simulink model "lqr_arduino_basic"  (R2015a)
settings: Solver=ode3  StartTime=0.0  StopTime=10.0  FixedStep=1/200  RelTol=1e-3
undefined symbols (not defined in the file or in its folder): Discrete, Hinf, Obs, Obs2, Time
libraries: PoliArd x8, ctrlSharedLib x2, simulink x1
settings Model: ExtModeTrigDuration=2  Creator=User  LastModifiedBy=user
settings OptimizationCC: OptimizeModelRefInitCode=on  LifeSpan=1
settings DebuggingCC: UnderspecifiedInitializationDetection=Classic  MergeDetectMultiDrivingBlocksExec=none
settings HardwareCC: ProdLargestAtomicInteger=Long  ProdLargestAtomicFloat=Double  ProdEndianess=LittleEndian  ProdHWDeviceType=ARM Compatible->ARM Cortex
settings RTWCC: SystemTargetFile=realtime.tlc  GenerateMakefile=off  TemplateMakefile=realtime.tmf  Description=Run on Target Hardware  RTWVerbose=off
settings ERTTargetCC: CombineOutputUpdateFcns=off  ExtModeTransport=3  ExtModeMexFile=ext_serial_win32_comm_rtt  ExtModeMexArgs=0 1 9600  ERTSrcFileBannerTemplate=realtime_code_template.cgt  ERTHdrFileBannerTemplate=realtime_code_template.cgt  ERTDataSrcFileTemplate=realtime_code_template.cgt  ERTDataHdrFileTemplate=realtime_code_template.cgt  ERTCustomFileTemplate=realtime_file_process.tlc

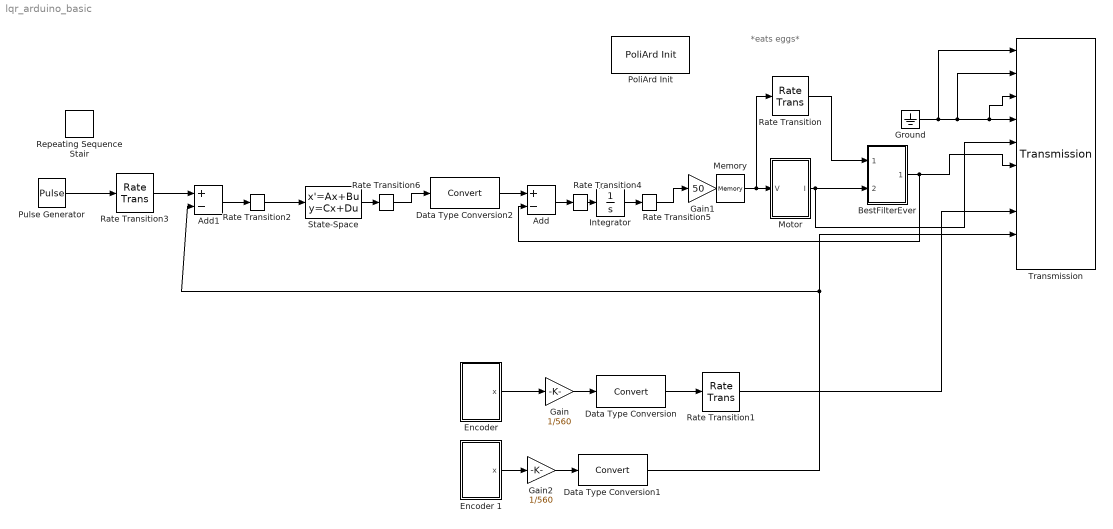
== system lqr_arduino_basic ==
  note: *eats eggs*
  Add : Sum  Inputs=+-
  Add1 : Sum  Inputs=+-
  BestFilterEver : Subsystem
  Data Type Conversion : DataTypeConversion
  Data Type Conversion1 : DataTypeConversion
  Data Type Conversion2 : DataTypeConversion
  "Encoder " : Subsystem
  Encoder 1 : Subsystem
  Gain : Gain  Gain=1/560
  Gain1 : Gain  Gain=50
  Gain2 : Gain  Gain=1/560
  Ground : Ground
  Integrator : Integrator
  Memory : Memory  InheritSampleTime=on
  Motor : Subsystem
  PoliArd Init : PoliArd/PoliArd Init
  Pulse Generator : DiscretePulseGenerator  PulseType=Time based  Amplitude=1.5  Period=7  PulseWidth=50  PhaseDelay=3
  Rate Transition{,1..6} (7 alike) : RateTransition
  Repeating Sequence Stair : simulink/Sources/Repeating Sequence Stair  OutValues=[1 2 -1 -2]  tsamp=5  OutMin=[]  OutMax=[]  OutDataTypeStr=double  OutputDataTypeScalingMode=double  OutDataType=fixdt(0,8)  ConRadixGroup=Best Precision: Vector-wise  OutScaling=2^-12
  State-Space : StateSpace  A=Hinf.A  B=Hinf.B  C=Hinf.C  D=Hinf.D  X0=0
  Transmission : PoliArd/Transmission  sample_freq=200  sig_to_send=6
  wires:
  Ground/1 -> Transmission/2, Transmission/3, Transmission/4, Transmission/1
  "Encoder "/1(x) -> Gain/1
  Gain/1 -> Data Type Conversion/1
  Data Type Conversion/1 -> Rate Transition1/1
  Encoder 1/1(x) -> Gain2/1
  Gain2/1 -> Data Type Conversion1/1
  Data Type Conversion1/1 -> Transmission/9, Add1/2
  Rate Transition1/1 -> Transmission/8
  Pulse Generator/1 -> Rate Transition3/1
  Motor/1(I) -> Transmission/5, BestFilterEver/2(In2)
  Rate Transition/1 -> BestFilterEver/1(In1)
  BestFilterEver/1(Out2) -> Add/2, Transmission/6
  Add/1 -> Rate Transition4/1
  Gain1/1 -> Memory/1
  Rate Transition5/1 -> Gain1/1
  Integrator/1 -> Rate Transition5/1
  Rate Transition4/1 -> Integrator/1
  Rate Transition3/1 -> Add1/1
  Add1/1 -> Rate Transition2/1
  Rate Transition2/1 -> State-Space/1
  State-Space/1 -> Rate Transition6/1
  Rate Transition6/1 -> Data Type Conversion2/1
  Data Type Conversion2/1 -> Add/1
  Memory/1 -> Rate Transition/1, Motor/1(V)

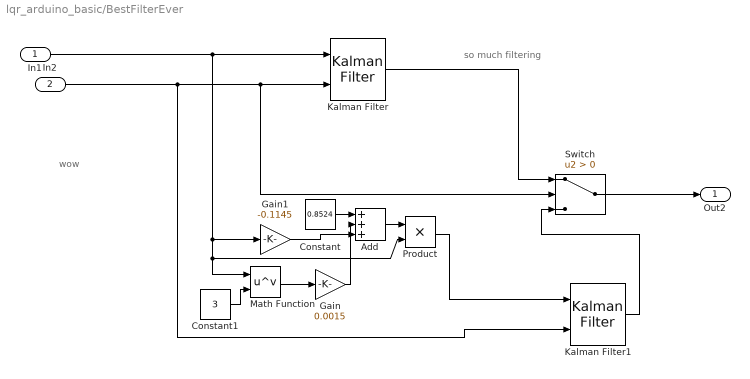
== system lqr_arduino_basic/BestFilterEver ==
  note: wow
  note: so much filtering
  In1 : Inport
  In2 : Inport  Port=2
  Add : Sum  Inputs=+++
  Constant : Constant  Value=0.8524
  Constant1 : Constant  Value=3
  Gain : Gain  Gain=0.0015
  Gain1 : Gain  Gain=-0.1145
  Kalman Filter : ctrlSharedLib/Kalman Filter  TimeDomain=Discrete-Time  UseCurrentEstimator=on  ModelSource=Individual A, B, C, D matrices  ModelSourceVariable=ss(0.95,1,1,0,1)  A=Obs.a  B=Obs.b  C=Obs.c  D=Obs.d  NumberOfStates=1  NumberOfInputs=1  NumberOfOutputs=1  InitialEstimateSource=Dialog  X0=0  P0=10  UseK=off  UseGH=off  NumberOfProcessNoiseInputs=1  G=1  TimeInvariantG=on  H=0  TimeInvariantH=on  Q=1e-9  TimeInvariantQ=on  R=0.0015  TimeInvariantR=on  N=0  TimeInvariantN=on  AddInputPort=on  AddEnablePort=off  OutputEstimatedY=off  OutputP=off  Ts=-1
  Kalman Filter1 : ctrlSharedLib/Kalman Filter  TimeDomain=Discrete-Time  UseCurrentEstimator=on  ModelSource=Individual A, B, C, D matrices  ModelSourceVariable=ss(0.95,1,1,0,1)  A=Obs2.a  B=Obs2.b  C=Obs2.c  D=Obs2.d  NumberOfStates=1  NumberOfInputs=1  NumberOfOutputs=1  InitialEstimateSource=Dialog  X0=0  P0=10  UseK=off  UseGH=off  NumberOfProcessNoiseInputs=1  G=1  TimeInvariantG=on  H=0  TimeInvariantH=on  Q=1e-9  TimeInvariantQ=on  R=0.0127  TimeInvariantR=on  N=0  TimeInvariantN=on  AddInputPort=on  AddEnablePort=off  OutputEstimatedY=off  OutputP=off  Ts=-1
  Math Function : Math  Operator=pow  SaturateOnIntegerOverflow=on
  Product : Product
  Switch : Switch  Criteria=u2 > Threshold
  Out2 : Outport
  wires:
  Kalman Filter/1 -> Switch/1
  Kalman Filter1/1 -> Switch/3
  In1/1 -> Kalman Filter/1, Gain1/1, Product/2, Math Function/1
  Product/1 -> Kalman Filter1/1
  Constant1/1 -> Math Function/2
  Math Function/1 -> Gain/1
  Constant/1 -> Add/1
  Gain/1 -> Add/2
  Add/1 -> Product/1
  Gain1/1 -> Add/3
  In2/1 -> Kalman Filter1/2, Switch/2, Kalman Filter/2
  Switch/1 -> Out2/1

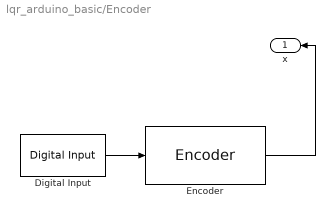
== system lqr_arduino_basic/Encoder  ==
  Digital Input : PoliArd/Digital Input  DI_pin=2  DIsample=1/200
  Encoder : PoliArd/Encoder  EncoderID=1  dt_enc=-1
  x : Outport
  wires:
  Digital Input/1 -> Encoder/1
  Encoder/1 -> x/1

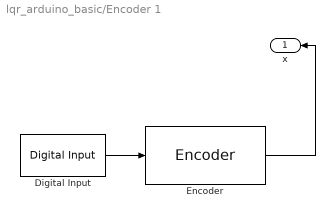
== system lqr_arduino_basic/Encoder 1 ==
  Digital Input : PoliArd/Digital Input  DI_pin=2  DIsample=1/200
  Encoder : PoliArd/Encoder  EncoderID=4  dt_enc=-1
  x : Outport
  wires:
  Digital Input/1 -> Encoder/1
  Encoder/1 -> x/1

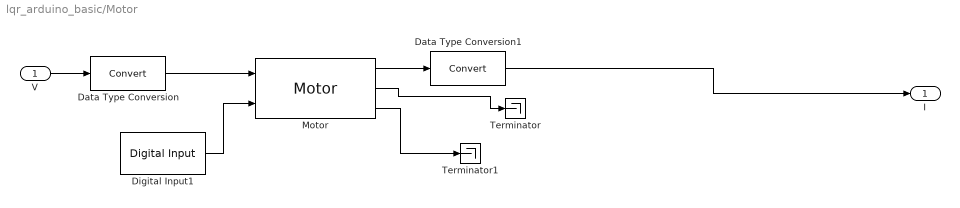
== system lqr_arduino_basic/Motor ==
  V : Inport
  Data Type Conversion : DataTypeConversion
  Data Type Conversion1 : DataTypeConversion
  Digital Input1 : PoliArd/Digital Input  DI_pin=3  DIsample=1/200
  Motor : PoliArd/Motor  MotorID=2  DC_bus_mask=12  dt_mot=1/200
  Terminator : Terminator
  Terminator1 : Terminator
  I : Outport
  wires:
  Data Type Conversion/1 -> Motor/1
  Digital Input1/1 -> Motor/2
  V/1 -> Data Type Conversion/1
  Motor/3 -> Terminator1/1
  Motor/2 -> Terminator/1
  Motor/1 -> Data Type Conversion1/1
  Data Type Conversion1/1 -> I/1
